simulink model "sampleModel1460"  (R2023a)
settings: Solver=VariableStepAuto  StartTime=0.0  StopTime=10.0  RelTol=1e-3
libraries: hdlsllib x4, simulink x3
settings Model: Creator=user1  LastModifiedBy=user1

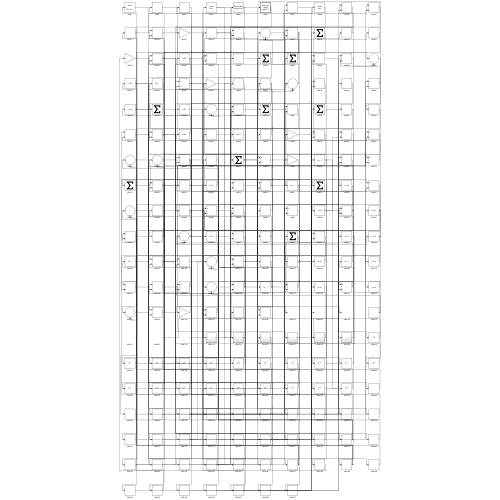
[thumbnail: Simulink's stored preview of the top-level diagram]
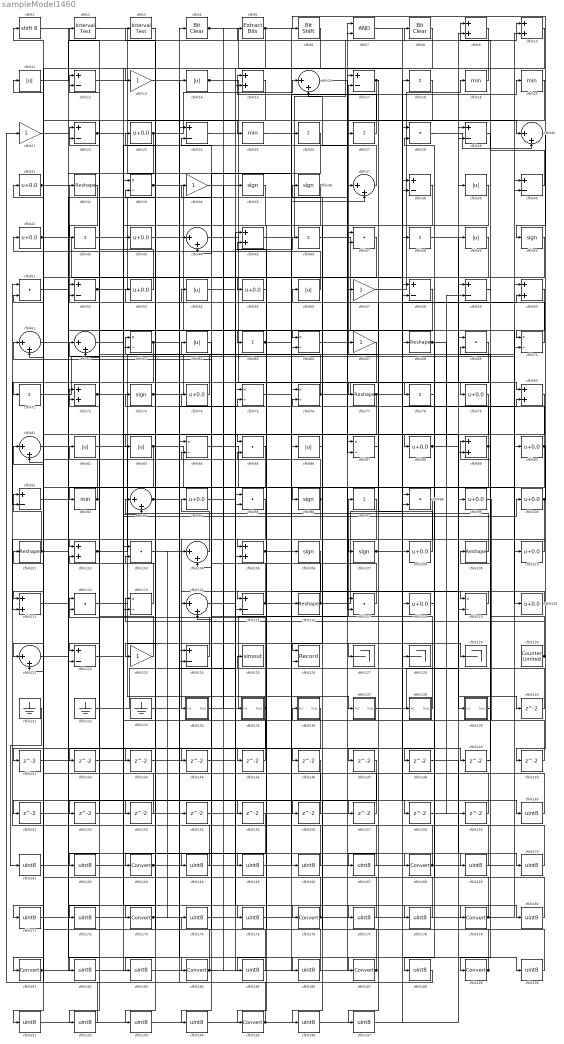
== system sampleModel1460 ==
  cfblk1 : ArithShift  BitShiftNumber=8
  cfblk{9..10,15,45,60,72,80,89,102,105,111} (11 alike) : Sum
  cfblk{23,31,41,43,53,55,74,79,88,90,94,99..100,108,110,118,120} (17 alike) : Bias  Bias=0.0  SaturateOnIntegerOverflow=off
  cfblk{32,68,77,101,109,116} (6 alike) : Reshape
  cfblk{28,47,51,69,85,95,98,103,112,117} (10 alike) : DotProduct  OutDataTypeStr=Inherit: Inherit via internal rule
  cfblk{16,30,37,44,61..62,81,93,104,114,121} (11 alike) : Sum  Inputs=|++
  cfblk{35..36,50,73,96,106..107} (7 alike) : Signum
  cfblk{11,14,39,49,54,56,64,82..83,86} (10 alike) : Abs  SaturateOnIntegerOverflow=off
  cfblk{33,63,66,70,75..76,84,87,113,119} (10 alike) : Product  Inputs=*/  RndMeth=Zero  SaturateOnIntegerOverflow=on
  cfblk{12,17,22,24,29,38,40,52,58..59,91,115,122,124} (14 alike) : Sum  Inputs=+-
  cfblk{13,21,34,57,67,123} (6 alike) : Gain
  cfblk125 : ToWorkspace  VariableName=simout  SaveFormat=Timeseries  SampleTime=-1
  cfblk126 : Record  FileSettingsInternal="{\"entries\":[{\"content\":{\"excelSettings\":{\"content\":{},\"type\":\"Streamout.ExcelSettings\"}},\"type\":\"Streamout.FileSettingStorage\",\"uuid\":\"\"}],\"packageUris\":[\"http:\\/\\/schema.mathworks.com\\/mf0\\/streamout_blocks\\/R2020a\"],\"version\":\"1.0\"}"  Layout=[1 1]  SignalsInternal="{\"entries\":[{\"content\":{\"signals\":[{\"content\":{\"blockPath\":[],\"dimensions\":[1],\"domain\":\"\",\"lineColor\":\"#a2142f\",\"plots\":[1],\"port\":1,\"signalID\":846,\"signalName\":\"XY Graph:1\"},\"type\":\"RecordBlkView.Signal\",\"uuid\":\"\"},{\"content\":{\"blockPath\":[],\"dimensions\":[1],\"domain\":\"\",\"lineColor\":\"#139fff\",\"plots\":[1],\"port\":2,\"signalID\":849,\"signalName\":\"XY Graph:2\"},\"type\":\"RecordBlkView.Signal\",\"uuid\":\"\"}]},\"type\":\"RecordBlkView.InputSignals\",\"uuid\":\"\"}],\"packageUris\":[\"http:\\/\\/schema.mathworks.com\\/mf0\\/streamout_blocks\\/R2020a\"],\"version\":\"1.0\"}"  VisualizationBindings="{\"xyplotplugin\":{\"info\":[{\"series\":[{\"bindingParametersList\":[{\"parameter\":\"X-Axis\",\"signalID\":846,\"signalName\":\"XY Graph:1\"},{\"parameter\":\"Y-Axis\",\"signalID\":849,\"signalName\":\"XY Graph:2\"}],\"seriesID\":27397}],\"subplotID\":1}]}}"  CompatibilityTag=XY  st=-1
  cfblk127 : Terminator
  cfblk128 : Terminator
  cfblk129 : Terminator
  cfblk130 : hdlsllib/Sources/Counter Limited  uplimit=7  tsamp=-1
  cfblk131 : Ground
  cfblk132 : Ground
  cfblk133 : Ground
  cfblk134 : Subsystem
      settings: LibrarySourceBlock=|
      | hdlsllib/Ports &
      | Subsystems/Subsystem
  cfblk135 : Subsystem
      settings: LibrarySourceBlock=|
      | hdlsllib/Ports &
      | Subsystems/Subsystem
  cfblk136 : Subsystem
      settings: LibrarySourceBlock=|
      | hdlsllib/Ports &
      | Subsystems/Subsystem
  cfblk137 : Subsystem
      settings: LibrarySourceBlock=|
      | hdlsllib/Ports &
      | Subsystems/Subsystem
  cfblk138 : Subsystem
      settings: LibrarySourceBlock=|
      | hdlsllib/Ports &
      | Subsystems/Subsystem
  cfblk139 : Subsystem
      settings: LibrarySourceBlock=|
      | hdlsllib/Ports &
      | Subsystems/Subsystem
  cfblk{140..159} (20 alike) : Delay  SampleTime=1
  cfblk{160..162,164..167,169..172,174..175,177..178,180,182..183,185..186,188,190..194,196..197} (28 alike) : DataTypeConversion  OutDataTypeStr=uint8  SaturateOnIntegerOverflow=off  RndMeth=Floor
  cfblk{163,168,173,176,179,181,184,187,189,195} (10 alike) : DataTypeConversion  SaturateOnIntegerOverflow=off  RndMeth=Floor
  cfblk{18,26..27,42,46,48,65,71,78,97} (10 alike) : Sum  Inputs=+
  cfblk{19..20,25,92} (4 alike) : MinMax
  cfblk2 : hdlsllib/Logic and Bit Operations/Interval Test  IntervalClosedRight=on  uplimit=0.5  IntervalClosedLeft=on  lowlimit=-0.5  OutDataTypeStr=boolean
  cfblk3 : hdlsllib/Logic and Bit Operations/Interval Test  IntervalClosedRight=on  uplimit=0.5  IntervalClosedLeft=on  lowlimit=-0.5  OutDataTypeStr=boolean
  cfblk4 : simulink/Logic and Bit Operations/Bit Clear  iBit=0
      settings: LibrarySourceBlock=|
      | hdlsllib/Logic and Bit
      | Operations/Bit Clear
  cfblk5 : simulink/Logic and Bit Operations/Extract Bits  bitsToExtract=Upper half  numBits=8  bitIdxRange=[0 7]  outScalingMode=Preserve fixed-point scaling
      settings: LibrarySourceBlock=|
      | hdlsllib/Logic and Bit
      | Operations/Extract Bits
  cfblk6 : hdlsllib/Logic and Bit Operations/Bit Shift  mode=Shift Left Logical  N=0
  cfblk7 : Logic  AllPortsSameDT=off  OutDataTypeStr=boolean
  cfblk8 : simulink/Logic and Bit Operations/Bit Clear  iBit=0
      settings: LibrarySourceBlock=|
      | hdlsllib/Logic and Bit
      | Operations/Bit Clear
  wires:
  cfblk119/1 -> cfblk115/1
  cfblk90/1 -> cfblk92/1, cfblk23/1, cfblk117/2, cfblk150/1
  cfblk23/1 -> cfblk16/1, cfblk122/2
  cfblk132/1 -> cfblk75/1
  cfblk102/1 -> cfblk64/1, cfblk100/1, cfblk180/1
  cfblk72/1 -> cfblk122/1, cfblk10/2, cfblk39/1
  cfblk139/1(Out1) -> cfblk109/1
  cfblk81/1 -> cfblk184/1
  cfblk112/1 -> cfblk127/1
  cfblk14/1 -> cfblk106/1, cfblk77/1
  cfblk66/1 -> cfblk17/2
  cfblk45/1 -> cfblk8/1
  cfblk117/1 -> cfblk63/1
  cfblk69/1 -> cfblk102/1
  cfblk16/1 -> cfblk30/1
  cfblk34/1 -> cfblk179/1
  cfblk60/1 -> cfblk70/1
  cfblk9/1 -> cfblk63/2
  cfblk99/1 -> cfblk136/1(In1)
  cfblk27/1 -> cfblk15/1
  cfblk115/1 -> cfblk26/1, cfblk74/1, cfblk54/1
  cfblk114/1 -> cfblk45/1
  cfblk21/1 -> cfblk187/1
  cfblk82/1 -> cfblk137/1(In1)
  cfblk83/1 -> cfblk139/1(In1), cfblk110/1, cfblk182/1
  cfblk28/1 -> cfblk30/2
  cfblk70/1 -> cfblk32/1
  cfblk47/1 -> cfblk173/1
  cfblk2/1 -> cfblk25/1
  cfblk8/1 -> cfblk83/1
  cfblk109/1 -> cfblk93/1
  cfblk89/1 -> cfblk121/1, cfblk67/1
  cfblk135/1(Out1) -> cfblk112/1, cfblk162/1
  cfblk98/1 -> cfblk134/1(In1)
  cfblk57/1 -> cfblk19/1
  cfblk88/1 -> cfblk59/2, cfblk140/1
  cfblk73/1 -> cfblk60/1, cfblk186/1
  cfblk41/1 -> cfblk55/1, cfblk66/2
  cfblk104/1 -> cfblk94/1
  cfblk12/1 -> cfblk116/1
  cfblk100/1 -> cfblk6/1, cfblk111/2
  cfblk52/1 -> cfblk4/1, cfblk89/2
  cfblk97/1 -> cfblk105/1
  cfblk33/1 -> cfblk120/1, cfblk158/1
  cfblk113/1 -> cfblk62/1
  cfblk31/1 -> cfblk96/1, cfblk156/1
  cfblk4/1 -> cfblk128/1, cfblk135/1(In1)
  cfblk17/1 -> cfblk87/2, cfblk142/1, cfblk197/1
  cfblk56/1 -> cfblk41/1
  cfblk75/1 -> cfblk20/1
  cfblk22/1 -> cfblk93/2, cfblk175/1
  cfblk32/1 -> cfblk42/1
  cfblk54/1 -> cfblk78/1
  cfblk93/1 -> cfblk14/1, cfblk75/2
  cfblk65/1 -> cfblk119/2, cfblk169/1
  cfblk124/1 -> cfblk12/1
  cfblk10/1 -> cfblk105/2
  cfblk92/1 -> cfblk11/1, cfblk72/1
  cfblk6/1 -> cfblk15/2
  cfblk91/1 -> cfblk112/2
  cfblk96/1 -> cfblk22/2, cfblk143/1
  cfblk120/1 -> cfblk114/1
  cfblk134/1(Out1) -> cfblk97/1
  cfblk71/1 -> cfblk40/1
  cfblk44/1 -> cfblk108/1
  cfblk37/1 -> cfblk16/2
  cfblk95/1 -> cfblk181/1
  cfblk55/1 -> cfblk85/1
  cfblk130/1 -> cfblk89/1, cfblk113/1
  cfblk68/1 -> cfblk88/1, cfblk159/1
  cfblk86/1 -> cfblk36/1
  cfblk29/1 -> cfblk189/1
  cfblk74/1 -> cfblk2/1
  cfblk77/1 -> cfblk80/2, cfblk164/1
  cfblk26/1 -> cfblk44/2
  cfblk85/1 -> cfblk124/2
  cfblk123/1 -> cfblk62/2
  cfblk138/1(Out1) -> cfblk61/1
  cfblk63/1 -> cfblk111/1, cfblk91/2, cfblk146/1
  cfblk116/1 -> cfblk68/1, cfblk73/1
  cfblk137/1(Out1) -> cfblk49/1
  cfblk43/1 -> cfblk66/1
  cfblk94/1 -> cfblk46/1
  cfblk53/1 -> cfblk22/1
  cfblk84/1 -> cfblk118/1
  cfblk39/1 -> cfblk126/1
  cfblk62/1 -> cfblk27/1
  cfblk50/1 -> cfblk71/1
  cfblk30/1 -> cfblk50/1
  cfblk24/1 -> cfblk176/1
  cfblk46/1 -> cfblk70/2
  cfblk19/1 -> cfblk13/1
  cfblk40/1 -> cfblk9/1
  cfblk59/1 -> cfblk119/1
  cfblk3/1 -> cfblk163/1
  cfblk108/1 -> cfblk57/1
  cfblk76/1 -> cfblk79/1, cfblk33/2
  cfblk20/1 -> cfblk52/2
  cfblk11/1 -> cfblk5/1
  cfblk133/1 -> cfblk10/1
  cfblk5/1 -> cfblk121/2, cfblk149/1
  cfblk48/1 -> cfblk80/1
  cfblk110/1 -> cfblk107/1
  cfblk101/1 -> cfblk37/1, cfblk91/1
  cfblk38/1 -> cfblk195/1
  cfblk105/1 -> cfblk37/2, cfblk129/1
  cfblk103/1 -> cfblk168/1
  cfblk36/1 -> cfblk123/1, cfblk113/2
  cfblk107/1 -> cfblk138/1(In1), cfblk60/2
  cfblk1/1 -> cfblk65/1
  cfblk140/1 -> cfblk124/1
  cfblk79/1 -> cfblk141/1
  cfblk141/1 -> cfblk115/2
  cfblk142/1 -> cfblk44/1
  cfblk106/1 -> cfblk144/1
  cfblk144/1 -> cfblk114/2
  cfblk111/1 -> cfblk145/1
  cfblk145/1 -> cfblk33/1
  cfblk80/1 -> cfblk147/1
  cfblk118/1 -> cfblk148/1
  cfblk149/1 -> cfblk69/2
  cfblk150/1 -> cfblk85/2
  cfblk136/1(Out1) -> cfblk151/1
  cfblk151/1 -> cfblk17/1
  cfblk15/1 -> cfblk152/1
  cfblk152/1 -> cfblk102/2
  cfblk35/1 -> cfblk153/1
  cfblk153/1 -> cfblk52/1
  cfblk154/1 -> cfblk76/1
  cfblk42/1 -> cfblk155/1
  cfblk156/1 -> cfblk12/2
  cfblk61/1 -> cfblk157/1
  cfblk157/1 -> cfblk45/2
  cfblk158/1 -> cfblk59/1
  cfblk159/1 -> cfblk1/1
  cfblk7/1 -> cfblk160/1
  cfblk160/1 -> cfblk82/1
  cfblk131/1 -> cfblk161/1
  cfblk161/1 -> cfblk7/1
  cfblk162/1 -> cfblk7/2
  cfblk163/1 -> cfblk126/2, cfblk87/1, cfblk90/1
  cfblk164/1 -> cfblk3/1
  cfblk51/1 -> cfblk165/1
  cfblk165/1 -> cfblk99/1
  cfblk25/1 -> cfblk166/1
  cfblk166/1 -> cfblk51/1
  cfblk87/1 -> cfblk167/1
  cfblk167/1 -> cfblk51/2
  cfblk168/1 -> cfblk9/2, cfblk56/1
  cfblk169/1 -> cfblk103/1
  cfblk148/1 -> cfblk170/1
  cfblk170/1 -> cfblk103/2
  cfblk18/1 -> cfblk171/1
  cfblk171/1 -> cfblk98/2
  cfblk67/1 -> cfblk172/1
  cfblk172/1 -> cfblk18/1
  cfblk173/1 -> cfblk154/1, cfblk104/1
  cfblk174/1 -> cfblk47/1
  cfblk175/1 -> cfblk47/2
  cfblk176/1 -> cfblk84/2, cfblk48/1, cfblk40/2
  cfblk121/1 -> cfblk177/1
  cfblk177/1 -> cfblk24/1
  cfblk122/1 -> cfblk178/1
  cfblk178/1 -> cfblk24/2
  cfblk179/1 -> cfblk28/2, cfblk61/2, cfblk98/1
  cfblk180/1 -> cfblk34/1
  cfblk181/1 -> cfblk72/2, cfblk43/1
  cfblk182/1 -> cfblk95/1
  cfblk143/1 -> cfblk183/1
  cfblk183/1 -> cfblk95/2
  cfblk184/1 -> cfblk174/1, cfblk117/1, cfblk35/1, cfblk86/1
  cfblk49/1 -> cfblk185/1
  cfblk185/1 -> cfblk81/1
  cfblk186/1 -> cfblk81/2
  cfblk187/1 -> cfblk104/2, cfblk53/1, cfblk101/1
  cfblk78/1 -> cfblk188/1
  cfblk188/1 -> cfblk21/1
  cfblk189/1 -> cfblk28/1, cfblk125/1, cfblk76/2
  cfblk13/1 -> cfblk190/1
  cfblk190/1 -> cfblk29/1
  cfblk146/1 -> cfblk191/1
  cfblk191/1 -> cfblk29/2
  cfblk58/1 -> cfblk192/1
  cfblk192/1 -> cfblk31/1
  cfblk155/1 -> cfblk193/1
  cfblk193/1 -> cfblk58/1
  cfblk64/1 -> cfblk194/1
  cfblk194/1 -> cfblk58/2
  cfblk195/1 -> cfblk84/1, cfblk69/1
  cfblk147/1 -> cfblk196/1
  cfblk196/1 -> cfblk38/1
  cfblk197/1 -> cfblk38/2

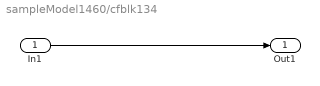
== system sampleModel1460/cfblk134 ==
  In1 : Inport
  Out1 : Outport
  wires:
  In1/1 -> Out1/1

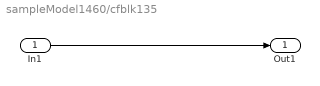
== system sampleModel1460/cfblk135 ==
  In1 : Inport
  Out1 : Outport
  wires:
  In1/1 -> Out1/1

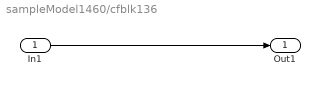
== system sampleModel1460/cfblk136 ==
  In1 : Inport
  Out1 : Outport
  wires:
  In1/1 -> Out1/1

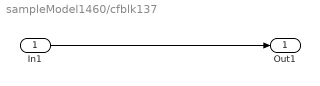
== system sampleModel1460/cfblk137 ==
  In1 : Inport
  Out1 : Outport
  wires:
  In1/1 -> Out1/1

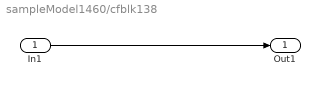
== system sampleModel1460/cfblk138 ==
  In1 : Inport
  Out1 : Outport
  wires:
  In1/1 -> Out1/1

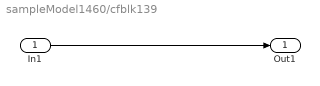
== system sampleModel1460/cfblk139 ==
  In1 : Inport
  Out1 : Outport
  wires:
  In1/1 -> Out1/1
